simulink model "Battery_sim_2"  (R2026a)
settings: Solver=FixedStepAuto  StopTime=n_years*8760  FixedStep=1
values from neighbouring files (symbols this model uses):
  a_montes = 0.869    [WS_Variables.mat]
  alpha_cal = 0.384    [WS_Variables.mat]
  bpC = [-0.25 -0.2 -0.15 -0.1 -0.05 0 0.05 0.1 0.15 0.2 0.25]    [WS_Variables.mat]
  bpSOC = [0 0.05 0.1 0.15 0.2 0.25 0.3 0.5 0.7 0.75 0.8 0.85 ... (15 elements, 15x1)]    [WS_Variables.mat]
  bpSOH = [0.8 0.9 1]    [WS_Variables.mat]
  dt_h = 1    [WS_Variables.mat]    (also in validate_fixes.m)
  Ea_cal = 20592    [WS_Variables.mat]
  eta_ch = 0.98    [WS_Variables.mat]
  eta_dis = 0.98    [WS_Variables.mat]
  F_const = 96485    [WS_Variables.mat]
  k0_cal = 0.142    [WS_Variables.mat]
  kcal_ref = 0.0003694    [WS_Variables.mat]
  kCch = 0.1038    [WS_Variables.mat]
  kCdch = 0.296    [WS_Variables.mat]
  kcyc = 0.003414    [WS_Variables.mat]
  kDODc = 0.0046    [WS_Variables.mat]
  kmSOC = 0.0513    [WS_Variables.mat]
  kT = 5.8755    [WS_Variables.mat]
  mapCeff = [0 0 0 0 0 0 0.0500000000002 0.1 0.149999999999 0.200000000001 0.249997995467 -0.00299426635782 ... (495 elements, 11x15x3)]    [WS_Variables.mat]
  mapTact = [0 0 0 0 0 0 1.00000000001 1.00000000001 1.00000000001 1.00000000001 1.00000000001 0.414516666666 ... (495 elements, 11x15x3)]    [WS_Variables.mat]
  mSOCref = 0.42    [WS_Variables.mat]
  Q_nom = 3    [WS_Variables.mat]
  R_ch_2D = [0.0536 0.0408 0.0368 0.0344 0.0288 0.0264 0.024 0.0595555555556 0.0453333333333 0.0408888888889 0.0382222222222 0.032 ... (77 elements, 7x11)]    [WS_Variables.mat]
  R_dis_2D = [0.1152 0.088 0.0768 0.072 0.064 0.0576 0.0528 0.0936 0.0715 0.0624 0.0585 0.052 ... (77 elements, 7x11)]    [WS_Variables.mat]
  R_gas = 8.314462618    [WS_Variables.mat]
  SOC0 = 0.5    [WS_Variables.mat]
  SOC_grid = [0 0.1 0.2 0.3 0.4 0.5 0.6 0.7 0.8 0.9 1]    [WS_Variables.mat]
  T_degC = 25    [WS_Variables.mat]
  T_grid_C = [10 20 25 30 40 50 60]    [WS_Variables.mat]
  Tref_cal = 298.15    [WS_Variables.mat]
  Tref_K = 298    [WS_Variables.mat]
  Ua_ref = 0.123    [WS_Variables.mat]
  V_nom = 3.2    [WS_Variables.mat]
undefined symbols (not defined in the file or in its folder): DiscIntNeverNeededParam
libraries: simulink x6
settings Model: Creator=Ali Khedr  LastModifiedBy=diaag
settings SimscapeCC: SimscapeNominalValues="[{\"value\":\"1\",\"unit\":\"A\"},{\"value\":\"1\",\"unit\":\"bar\"},{\"value\":\"1\",\"unit\":\"cm^2\"},{\"value\":\"1\",\"unit\":\"cm^3/s\"},{\"value\":\"1\",\"unit\":\"kJ/kg\"},{\"value\":\"1\",\"unit\":\"kW\"},{\"value\":\"1\",\"unit\":\"l\"},{\"value\":\"1\",\"unit\":\"N\"},{\"value\":\"1\",\"unit\":\"N*m\"},{\"value\":\"1\",\"unit\":\"V\"}]"  SimscapeLogType=none  SimscapeLogDataHistory=5000.0

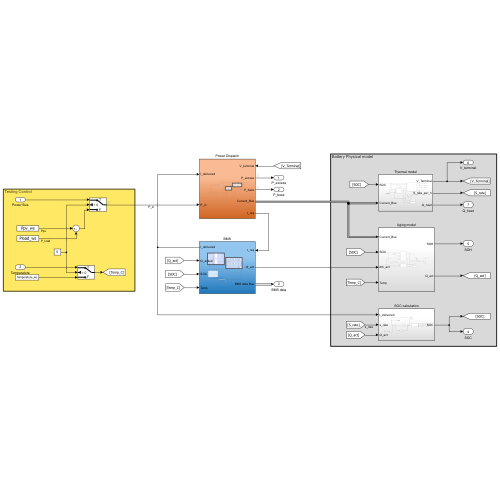
[thumbnail: Simulink's stored preview of the top-level diagram]
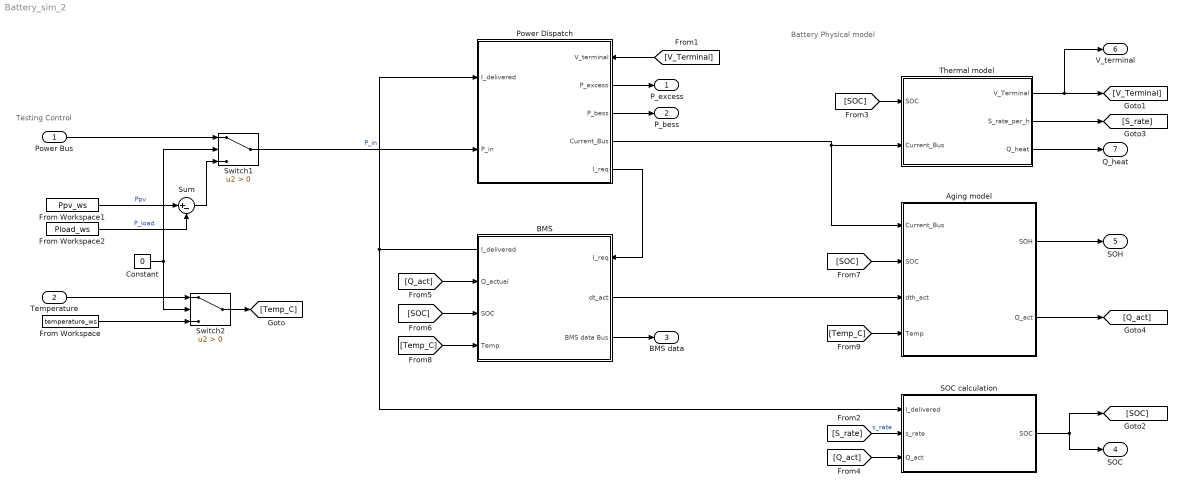
== system Battery_sim_2 ==
  note: Testing Control
  note: Battery Physical model
  Power Bus : Inport
  Temperature : Inport  Port=2
  Aging model : Subsystem
  BMS : Subsystem
      settings: PortSchema="{\"entries\":[{\"content\":{\"sides\":[{\"content\":{\"connectorIds\":[\"In1\",\"Out2\",\"Out3\"]},\"type\":\"ConnectorPlacement.EquallySpacedRectSide\",\"uuid\":\"b0358f3e-70d2-4a9b-a6b5-6f8f3d4044b9\"},{\"content\":{\"connectorIds\":[\"Out1\",\"In2\",\"In3\",\"In4\"],\"side\":\"RIGHT\"},\"type\":\"ConnectorPlacement.EquallySpacedRectSide\",\"uuid\":\"7236fea0-b457-4ecc-99f8-f1352261851b\"},{\"content\":{\"side\":\"TOP\"},\"type\":\"ConnectorPlacement.EquallySpacedRectSide\",\"uuid\":\"a18fdbf6-41d8-4990-8a17-1b53f0b4af4f\"},{\"content\":{\"side\":\"BOTTOM\"},\"type\":\"ConnectorPlacement.EquallySpacedRectSide\",\"uuid\":\"9a35465f-24db-4158-a547-c5af1beda424\"}]},\"type\":\"ConnectorPlacement.EquallySpacedConnector\",\"uuid\":\"ad446661-162d-463d-98d0-534800ba2a51\"}],\"packageUris\":[\"http://schema.mathworks.com/mf0/Connector/R2020b\"],\"version\":\"1.0\"}"
  Constant : Constant  Value=0
  From Workspace : FromWorkspace  VariableName=temperature_ws
  From Workspace1 : FromWorkspace  VariableName=Ppv_ws
  From Workspace2 : FromWorkspace  VariableName=Pload_ws
  Power Dispatch : Subsystem
      settings: PortSchema="{\"entries\":[{\"content\":{\"sides\":[{\"content\":{\"connectorIds\":[\"In1\",\"In2\"]},\"type\":\"ConnectorPlacement.EquallySpacedRectSide\",\"uuid\":\"ee44d7aa-69cc-41bc-9d41-e2128c2b3508\"},{\"content\":{\"connectorIds\":[\"In3\",\"Out1\",\"Out2\",\"Out3\",\"Out4\"],\"side\":\"RIGHT\"},\"type\":\"ConnectorPlacement.EquallySpacedRectSide\",\"uuid\":\"1a9a3f28-b2ae-47b5-968c-66d48cb4930a\"},{\"content\":{\"side\":\"TOP\"},\"type\":\"ConnectorPlacement.EquallySpacedRectSide\",\"uuid\":\"e022eaf0-aade-45fe-ae60-29b950c5dc81\"}]},\"type\":\"ConnectorPlacement.EquallySpacedConnector\",\"uuid\":\"4ff2f9de-87da-4d92-bb97-59c5bfa738bf\"}],\"packageUris\":[\"http://schema.mathworks.com/mf0/Connector/R2020b\"],\"version\":\"1.0\"}"
  SOC calculation : Subsystem
  Sum : Sum  Inputs=|+-
  Switch1 : Switch  Criteria=u2 > Threshold  SaturateOnIntegerOverflow=off  InputSameDT=off
  Switch2 : Switch  Criteria=u2 > Threshold  SaturateOnIntegerOverflow=off  InputSameDT=off
  Thermal model : Subsystem
  P_excess : Outport
  P_bess : Outport  Port=2
  BMS data : Outport  Port=3
  SOC : Outport  Port=4
  SOH : Outport  Port=5
  V_terminal : Outport  Port=6
  Q_heat : Outport  Port=7
  wires:
  Aging model/1(SOH) -> SOH/1
  Aging model/2(Q_act) -> [Q_act]
  [SOC] -> Thermal model/1(SOC)
  Thermal model/1(V_Terminal) -> [V_Terminal], V_terminal/1
  Thermal model/2(S_rate_per_h) -> [S_rate]
  BMS/2(dt_act) -> Aging model/3(dth_act)
  [Q_act] -> BMS/2(Q_actual)
  BMS/1(I_delivered) -> Power Dispatch/1(I_delivered), SOC calculation/1(I_delivered)
  Power Dispatch/3(Current_Bus) -> Aging model/1(Current_Bus), Thermal model/2(Current_Bus)
  [V_Terminal] -> Power Dispatch/3(V_terminal)
  Power Dispatch/4(I_req) -> BMS/1(I_req)
  [S_rate] -> SOC calculation/2(s_rate)  "s_rate"
  [Q_act] -> SOC calculation/3(Q_act)
  SOC calculation/1(SOC) -> SOC/1, [SOC]
  [SOC] -> BMS/3(SOC)
  [Temp_C] -> Aging model/4(Temp)
  [SOC] -> Aging model/2(SOC)
  Power Dispatch/1(P_excess) -> P_excess/1
  Power Dispatch/2(P_bess) -> P_bess/1
  BMS/3(BMS data Bus) -> BMS data/1
  Switch1/1 -> Power Dispatch/2(P_in)  "P_in"
  Constant/1 -> Switch1/2, Switch2/2
  Power Bus/1 -> Switch1/1
  From Workspace2/1 -> Sum/2  "P_load"
  From Workspace1/1 -> Sum/1  "Ppv"
  Sum/1 -> Switch1/3
  From Workspace/1 -> Switch2/3
  Temperature/1 -> Switch2/1
  Switch2/1 -> [Temp_C]
  [Temp_C] -> BMS/4(Temp)
  Thermal model/3(Q_heat) -> Q_heat/1

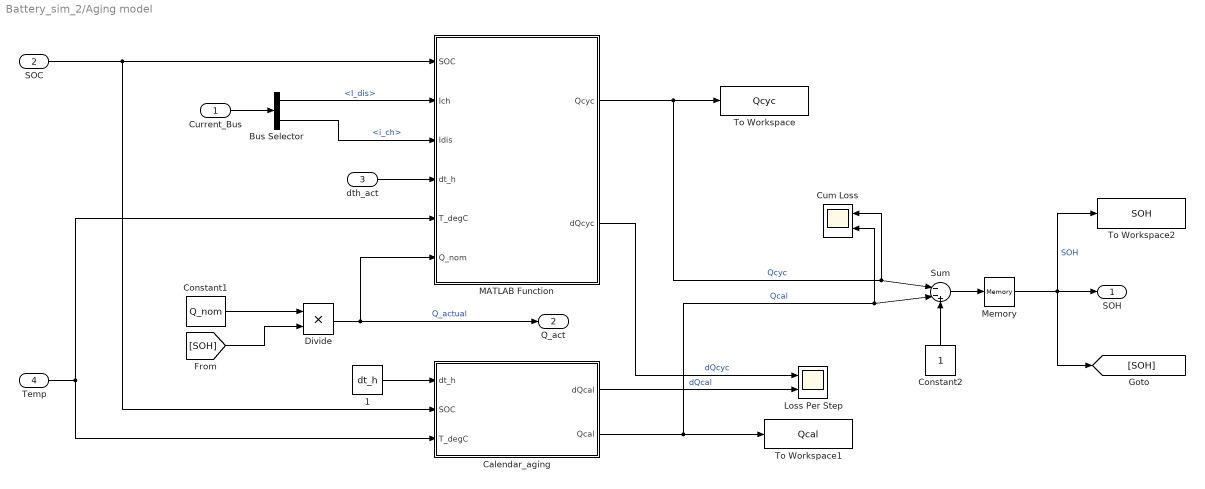
== system Battery_sim_2/Aging model ==
  Current_Bus : Inport
  SOC : Inport  Port=2
  dth_act : Inport  Port=3
  Temp : Inport  Port=4
  " 1" : Constant  Value=dt_h
  Bus Selector : BusSelector  OutputSignals=I_dis,i_ch
  Calendar_aging : Subsystem
  Constant1 : Constant  Value=Q_nom
  Constant2 : Constant
  Cum Loss : Scope  NumInputPorts=2
      settings: ActiveDisplayYMinimum=-0.04665783125845889  ActiveDisplayYMaximum=0.19177623612010322  DataLoggingVariableName=ScopeData5
  Divide : Product  Inputs=**
  Loss Per Step : Scope  NumInputPorts=2
      settings: ActiveDisplayYMinimum=-1.9153240746537514E-5  ActiveDisplayYMaximum=0.00017237916671883764
  MATLAB Function : MATLAB Function  TreatAsAtomicUnit=on
  Memory : Memory  InitialCondition=1
  Sum : Sum  Inputs=|--+
  To Workspace : ToWorkspace  VariableName=Qcyc  SaveFormat=Timeseries  SampleTime=-1
  To Workspace1 : ToWorkspace  VariableName=Qcal  SaveFormat=Timeseries  SampleTime=-1
  To Workspace2 : ToWorkspace  VariableName=SOH  SaveFormat=Timeseries  SampleTime=-1
  SOH : Outport
  Q_act : Outport  Port=2
  wires:
  MATLAB Function/2(dQcyc) -> Loss Per Step/1  "dQcyc"
  Temp/1 -> Calendar_aging/3(T_degC), MATLAB Function/5(T_degC)
  Calendar_aging/2(Qcal) -> To Workspace1/1, Sum/2, Cum Loss/2  "Qcal"
  Constant1/1 -> Divide/1
  Divide/1 -> MATLAB Function/6(Q_nom), Q_act/1  "Q_actual"
  MATLAB Function/1(Qcyc) -> Sum/1, Cum Loss/1, To Workspace/1  "Qcyc"
  Calendar_aging/1(dQcal) -> Loss Per Step/2  "dQcal"
  [SOH] -> Divide/2
  Sum/1 -> Memory/1
  Memory/1 -> [SOH], To Workspace2/1, SOH/1  "SOH"
  Constant2/1 -> Sum/3
  SOC/1 -> MATLAB Function/1(SOC), Calendar_aging/2(SOC)
  dth_act/1 -> MATLAB Function/4(dt_h)
  " 1"/1 -> Calendar_aging/1(dt_h)
  Current_Bus/1 -> Bus Selector/1
  Bus Selector/2 -> MATLAB Function/3(Idis)  "<i_ch>"
  Bus Selector/1 -> MATLAB Function/2(Ich)  "<I_dis>"

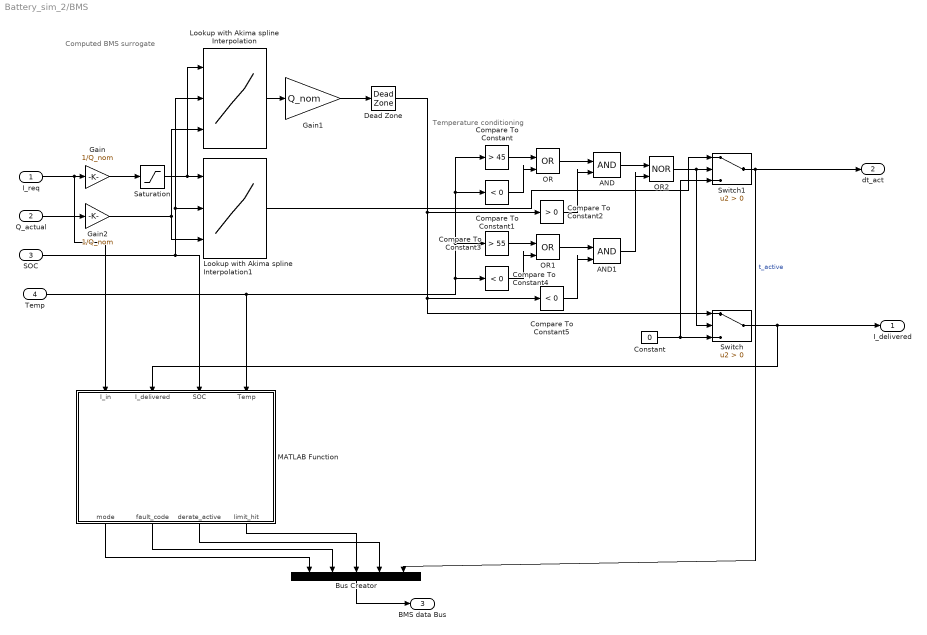
== system Battery_sim_2/BMS ==
  note: Temperature conditioning
  note: Computed BMS surrogate
  I_req : Inport
  Q_actual : Inport  Port=2
  SOC : Inport  Port=3
  Temp : Inport  Port=4
  AND : Logic  IconShape=distinctive  AllPortsSameDT=off  OutDataTypeStr=boolean
  AND1 : Logic  IconShape=distinctive  AllPortsSameDT=off  OutDataTypeStr=boolean
  Bus Creator : BusCreator  Inputs=5  OutDataTypeStr=Bus: BMS_Status  NonVirtualBus=on
      settings: InheritFromInputs=off
  Compare To Constant : simulink/Logic and Bit Operations/Compare To Constant  relop=>  const=45  OutDataTypeStr=boolean
  Compare To Constant1 : simulink/Logic and Bit Operations/Compare To Constant  relop=<  const=0  OutDataTypeStr=boolean
  Compare To Constant2 : simulink/Logic and Bit Operations/Compare To Constant  relop=>  const=0  OutDataTypeStr=boolean
  Compare To Constant3 : simulink/Logic and Bit Operations/Compare To Constant  relop=>  const=55  OutDataTypeStr=boolean
  Compare To Constant4 : simulink/Logic and Bit Operations/Compare To Constant  relop=<  const=0  OutDataTypeStr=boolean
  Compare To Constant5 : simulink/Logic and Bit Operations/Compare To Constant  relop=<  const=0  OutDataTypeStr=boolean
  Constant : Constant  Value=0
  Dead Zone : DeadZone  LowerValue=-0.01  UpperValue=0.0
  Gain : Gain  Gain=1/Q_nom
  Gain1 : Gain  Gain=Q_nom
  Gain2 : Gain  Gain=1/Q_nom
  Lookup with Akima spline Interpolation : Lookup_n-D  NumberOfTableDimensions=3  BreakpointsForDimension1=bpC  BreakpointsForDimension2=bpSOC  BreakpointsForDimension3=bpSOH  BreakpointsForDimension1DataTypeStr=double  BreakpointsForDimension2DataTypeStr=double  BreakpointsForDimension3DataTypeStr=double  Table=mapCeff  TableDataTypeStr=double  IntermediateResultsDataTypeStr=double  InternalRulePriority=Speed  OutDataTypeStr=double  RndMeth=Simplest  FractionDataTypeStr=double  InputSameDT=off
      settings: InputPortMap=u0,u1,u2
  Lookup with Akima spline Interpolation1 : Lookup_n-D  NumberOfTableDimensions=3  BreakpointsForDimension1=bpC  BreakpointsForDimension2=bpSOC  BreakpointsForDimension3=bpSOH  Table=mapTact  InterpMethod=Linear Lagrange  InternalRulePriority=Speed  OutDataTypeStr=double  RndMeth=Simplest
      settings: InputPortMap=u0,u1,u2
  MATLAB Function : MATLAB Function  TreatAsAtomicUnit=on
  OR : Logic  Operator=OR  IconShape=distinctive  AllPortsSameDT=off  OutDataTypeStr=boolean
  OR1 : Logic  Operator=OR  IconShape=distinctive  AllPortsSameDT=off  OutDataTypeStr=boolean
  OR2 : Logic  Operator=NOR  IconShape=distinctive  AllPortsSameDT=off  OutDataTypeStr=boolean
  Saturation : Saturate  UpperLimit=0.25  LowerLimit=-0.25
  Switch : Switch  Criteria=u2 > Threshold  SaturateOnIntegerOverflow=off  InputSameDT=off
  Switch1 : Switch  Criteria=u2 > Threshold  SaturateOnIntegerOverflow=off  InputSameDT=off
  I_delivered : Outport
  dt_act : Outport  Port=2
  BMS data Bus : Outport  Port=3  OutDataTypeStr=Bus: BMS_Status
  wires:
  Compare To Constant/1 -> OR/1
  Compare To Constant1/1 -> OR/2
  Compare To Constant5/1 -> AND1/2
  Compare To Constant4/1 -> OR1/2
  Compare To Constant3/1 -> OR1/1
  OR/1 -> AND/1
  Compare To Constant2/1 -> AND/2
  OR1/1 -> AND1/1
  AND/1 -> OR2/1
  AND1/1 -> OR2/2
  OR2/1 -> Switch1/2, Switch/2
  Constant/1 -> Switch1/3, Switch/3
  Gain/1 -> Saturation/1
  Saturation/1 -> Lookup with Akima spline Interpolation1/1, Lookup with Akima spline Interpolation/1
  Gain2/1 -> Lookup with Akima spline Interpolation/3, Lookup with Akima spline Interpolation1/3
  Gain1/1 -> Dead Zone/1
  Lookup with Akima spline Interpolation/1 -> Gain1/1
  Dead Zone/1 -> Compare To Constant2/1, Compare To Constant5/1, Switch/1
  SOC/1 -> MATLAB Function/3(SOC), Lookup with Akima spline Interpolation/2, Lookup with Akima spline Interpolation1/2
  Temp/1 -> Compare To Constant3/1, Compare To Constant1/1, Compare To Constant/1, Compare To Constant4/1, MATLAB Function/4(Temp)
  Switch1/1 -> Bus Creator/5, dt_act/1  "t_active"
  Lookup with Akima spline Interpolation1/1 -> Switch1/1
  I_req/1 -> MATLAB Function/1(I_in), Gain/1
  Q_actual/1 -> Gain2/1
  Switch/1 -> I_delivered/1, MATLAB Function/2(I_delivered)
  Bus Creator/1 -> BMS data Bus/1
  MATLAB Function/1(mode) -> Bus Creator/1
  MATLAB Function/2(fault_code) -> Bus Creator/2
  MATLAB Function/4(limit_hit) -> Bus Creator/3
  MATLAB Function/3(derate_active) -> Bus Creator/4

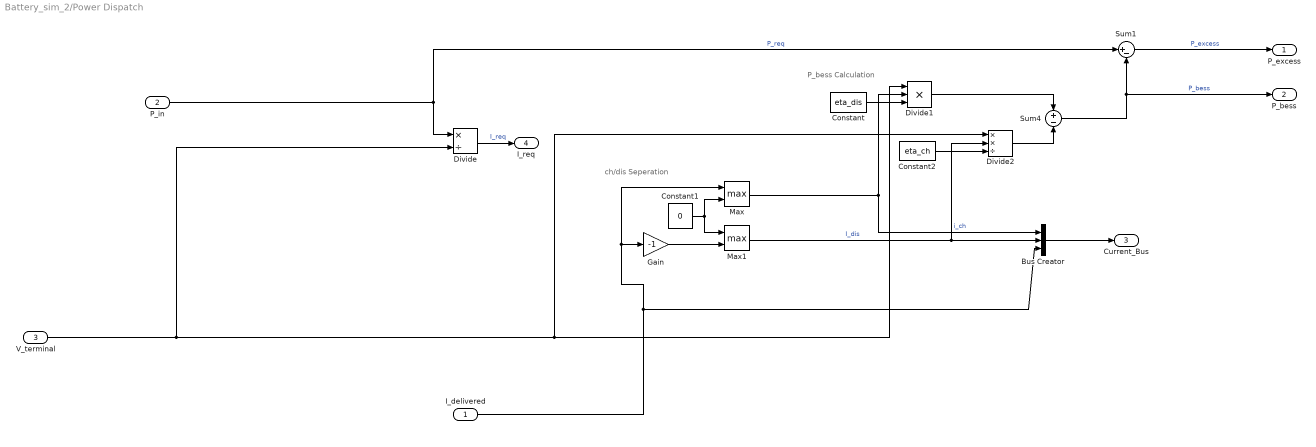
== system Battery_sim_2/Power Dispatch ==
  note: ch/dis Seperation
  note: P_bess Calculation
  I_delivered : Inport
  P_in : Inport  Port=2
  V_terminal : Inport  Port=3
  Bus Creator : BusCreator  Inputs=3
  Constant : Constant  Value=eta_dis
  Constant1 : Constant  Value=0
  Constant2 : Constant  Value=eta_ch
  Divide : Product  Inputs=*/
  Divide1 : Product  Inputs=***
  Divide2 : Product  Inputs=**/
  Gain : Gain  Gain=-1
  Max : MinMax  Function=max  Inputs=2
  Max1 : MinMax  Function=max  Inputs=2
  Sum1 : Sum  Inputs=|+-
  Sum4 : Sum  Inputs=+-
  P_excess : Outport
  P_bess : Outport  Port=2
  Current_Bus : Outport  Port=3
  I_req : Outport  Port=4
  wires:
  Sum4/1 -> Sum1/2, P_bess/1  "P_bess"
  V_terminal/1 -> Divide2/1, Divide1/1, Divide/2
  Max/1 -> Divide1/2, Bus Creator/1  "i_ch"
  Bus Creator/1 -> Current_Bus/1
  Divide2/1 -> Sum4/2
  Gain/1 -> Max1/2
  Divide1/1 -> Sum4/1
  Constant1/1 -> Max/2, Max1/1
  Constant2/1 -> Divide2/3
  Constant/1 -> Divide1/3
  P_in/1 -> Divide/1, Sum1/1  "P_req"
  Max1/1 -> Divide2/2, Bus Creator/2  "I_dis"
  I_delivered/1 -> Max/1, Gain/1, Bus Creator/3
  Divide/1 -> I_req/1  "I_req"
  Sum1/1 -> P_excess/1  "P_excess"

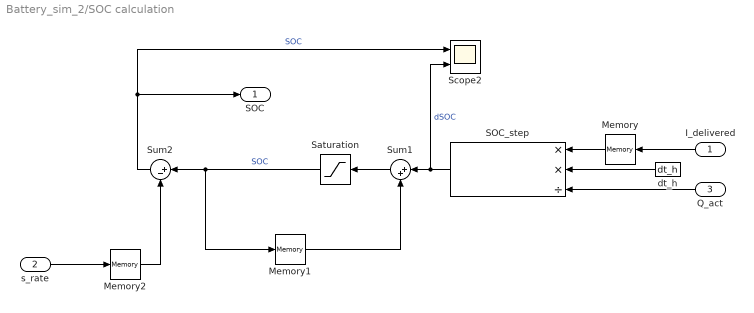
== system Battery_sim_2/SOC calculation ==
  I_delivered : Inport
  s_rate : Inport  Port=2
  Q_act : Inport  Port=3
  Memory : Memory
  Memory1 : Memory  InitialCondition=SOC0
  Memory2 : Memory
  SOC_step : Product  Inputs=**/
  Saturation : Saturate  UpperLimit=1  LowerLimit=0
  Scope2 : Scope  NumInputPorts=2
      settings: ActiveDisplayYMinimum=-0.083070549676689615  ActiveDisplayYMaximum=1.090372335178712  DataLoggingVariableName=ScopeData4
  Sum1 : Sum  Inputs=|++
  Sum2 : Sum  Inputs=|+-
  dt_h : Constant  Value=dt_h
  SOC : Outport
  wires:
  Memory/1 -> SOC_step/1
  Sum2/1 -> SOC/1, Scope2/1  "SOC"
  Memory1/1 -> Sum1/2
  SOC_step/1 -> Sum1/1, Scope2/2  "dSOC"
  Sum1/1 -> Saturation/1
  Saturation/1 -> Memory1/1, Sum2/1  "SOC"
  s_rate/1 -> Memory2/1
  dt_h/1 -> SOC_step/2
  Memory2/1 -> Sum2/2
  Q_act/1 -> SOC_step/3
  I_delivered/1 -> Memory/1

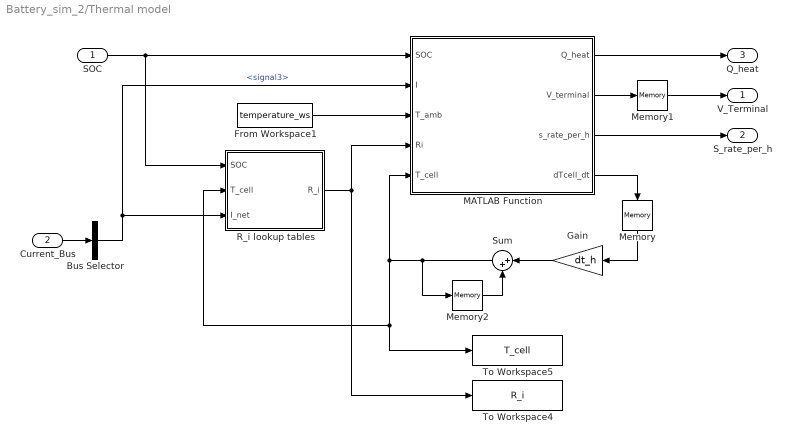
== system Battery_sim_2/Thermal model ==
  SOC : Inport
  Current_Bus : Inport  Port=2
  Bus Selector : BusSelector  OutputSignals=signal3
  From Workspace1 : FromWorkspace  VariableName=temperature_ws
  Gain : Gain  Gain=dt_h
  MATLAB Function : MATLAB Function  TreatAsAtomicUnit=on
  Memory : Memory
  Memory1 : Memory  InitialCondition=V_nom
  Memory2 : Memory  InitialCondition=T_degC
  R_i lookup tables : Subsystem
  Sum : Sum  Inputs=|++
  To Workspace4 : ToWorkspace  VariableName=R_i  SaveFormat=Timeseries  SampleTime=-1
  To Workspace5 : ToWorkspace  VariableName=T_cell  SaveFormat=Timeseries  SampleTime=-1
  V_Terminal : Outport
  S_rate_per_h : Outport  Port=2
  Q_heat : Outport  Port=3
  wires:
  Current_Bus/1 -> Bus Selector/1
  SOC/1 -> R_i lookup tables/1(SOC), MATLAB Function/1(SOC)
  From Workspace1/1 -> MATLAB Function/3(T_amb)
  MATLAB Function/2(V_terminal) -> Memory1/1
  MATLAB Function/4(dTcell_dt) -> Memory/1
  Memory/1 -> Gain/1
  Sum/1 -> To Workspace5/1, R_i lookup tables/2(T_cell), MATLAB Function/5(T_cell), Memory2/1
  Gain/1 -> Sum/1
  Memory2/1 -> Sum/2
  MATLAB Function/3(s_rate_per_h) -> S_rate_per_h/1
  R_i lookup tables/1(R_i) -> MATLAB Function/4(Ri), To Workspace4/1
  Memory1/1 -> V_Terminal/1
  Bus Selector/1 -> MATLAB Function/2(I), R_i lookup tables/3(I_net)  "<signal3>"
  MATLAB Function/1(Q_heat) -> Q_heat/1

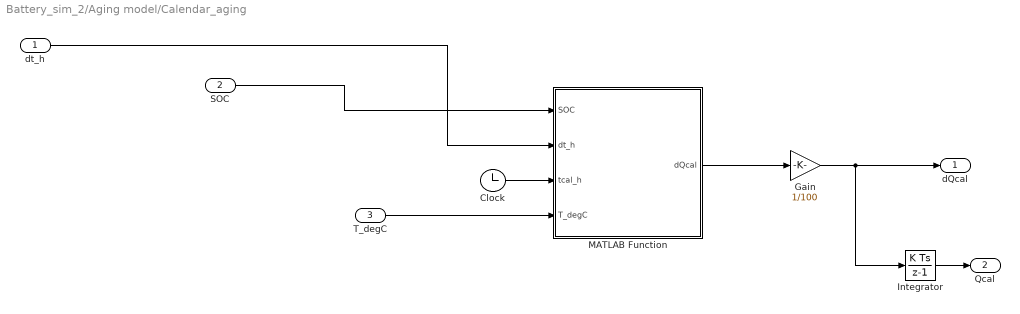
== system Battery_sim_2/Aging model/Calendar_aging ==
  dt_h : Inport
  SOC : Inport  Port=2
  T_degC : Inport  Port=3
  Clock : Clock
  Gain : Gain  Gain=1/100
  Integrator : DiscreteIntegrator  ICPrevOutput=DiscIntNeverNeededParam  ICPrevScaledInput=DiscIntNeverNeededParam
  MATLAB Function : MATLAB Function  TreatAsAtomicUnit=on
  dQcal : Outport
  Qcal : Outport  Port=2
  wires:
  SOC/1 -> MATLAB Function/1(SOC)
  Clock/1 -> MATLAB Function/3(tcal_h)
  dt_h/1 -> MATLAB Function/2(dt_h)
  MATLAB Function/1(dQcal) -> Gain/1
  T_degC/1 -> MATLAB Function/4(T_degC)
  Gain/1 -> dQcal/1, Integrator/1
  Integrator/1 -> Qcal/1

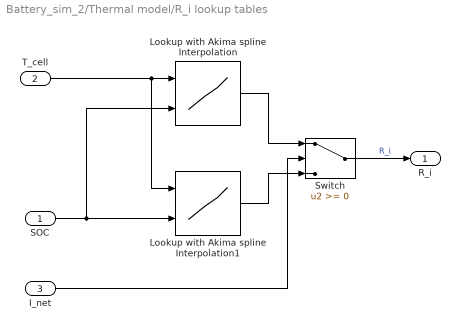
== system Battery_sim_2/Thermal model/R_i lookup tables ==
  SOC : Inport
  T_cell : Inport  Port=2
  I_net : Inport  Port=3
  Lookup with Akima spline Interpolation : Lookup_n-D  BreakpointsForDimension1=T_grid_C  BreakpointsForDimension2=SOC_grid  Table=R_ch_2D  InterpMethod=Akima spline  InternalRulePriority=Speed  RndMeth=Simplest
      settings: InputPortMap=u0,u1
  Lookup with Akima spline Interpolation1 : Lookup_n-D  BreakpointsForDimension1=T_grid_C  BreakpointsForDimension2=SOC_grid  Table=R_dis_2D  InterpMethod=Akima spline  InternalRulePriority=Speed  RndMeth=Simplest
      settings: InputPortMap=u0,u1
  Switch : Switch  SaturateOnIntegerOverflow=off  InputSameDT=off
  R_i : Outport
  wires:
  Lookup with Akima spline Interpolation/1 -> Switch/1
  Switch/1 -> R_i/1  "R_i"
  SOC/1 -> Lookup with Akima spline Interpolation/2, Lookup with Akima spline Interpolation1/2
  Lookup with Akima spline Interpolation1/1 -> Switch/3
  I_net/1 -> Switch/2
  T_cell/1 -> Lookup with Akima spline Interpolation1/1, Lookup with Akima spline Interpolation/1

== matlab function Battery_sim_2/Aging model/Calendar_aging/MATLAB Function ==
  data: SOC input; dQcal output; dt_h input; tcal_h input; T_degC input; Ea_cal parameter; R_gas parameter; Tref_cal parameter; alpha_cal parameter; F_const parameter; Ua_ref parameter; k0_cal parameter; kcal_ref parameter
function dQcal = calendar_aging(SOC, dt_h, tcal_h, T_degC, ...
    Ea_cal, R_gas, Tref_cal, alpha_cal, F_const, Ua_ref, k0_cal, kcal_ref)

dQcal = calendar_aging(SOC, dt_h, tcal_h, T_degC, ...
    Ea_cal, R_gas, Tref_cal, alpha_cal, F_const, Ua_ref, k0_cal, kcal_ref);
end

== matlab function Battery_sim_2/BMS/MATLAB Function ==
  settings: updateMethod=DISCRETE
  data: I_in input; I_delivered input; SOC input; mode output; Temp input; fault_code output; derate_active output boolean; limit_hit output
function [mode, fault_code, derate_active, limit_hit] = bms_status(I_in, I_delivered, SOC, Temp)
  cfg = bms_config();
  idle = cfg.mode.I_idle_thr;

  charging    = I_delivered >  idle;
  discharging = I_delivered < -idle;

  reduced = abs(I_delivered) < abs(I_in) - idle;          % limited but flowing
  cut     = (abs(I_in) > idle) && (abs(I_delivered) <= idle);  % fully blocked

  % why it was blocked (instantaneous, no latch)
  cold  = (Temp < cfg.cell.T_chg_min);
  hot   = (charging && Temp > cfg.cell.T_chg_max) || (discharging && Temp > cfg.cell.T_dis_max);
  soclim = (charging && SOC >= cfg.soc.window_max) || (discharging && SOC <= cfg.soc.window_min);

  fault_code = 0;                       % 0 none
  if cut
      if cold,  fault_code = 1;         % cold-charge block
      elseif hot, fault_code = 2;       % over-temp block
      elseif soclim, fault_code = 3;    % SOC floor/ceiling
      else 
          fault_code = 4; end          % other (request cut for another reason)
  end

  derate_active = reduced && ~cut;
  limit_hit     = cut;

  if cut,               mode = cfg.mode.FAULT;
  elseif derate_active, mode = cfg.mode.DERATE;
  elseif charging,      mode = cfg.mode.CHARGE;
  elseif discharging,   mode = cfg.mode.DISCHARGE;
  else                  mode = cfg.mode.STANDBY;
  end
end

== matlab function Battery_sim_2/Aging model/MATLAB Function ==
  settings: updateMethod=DISCRETE
  data: SOC input; Qcyc output; Ich input; Idis input; dt_h input; T_degC input; Q_nom input; kT parameter; Tref_K parameter; kDODc parameter; kcyc parameter; kCch parameter; kCdch parameter; kmSOC parameter; mSOCref parameter; a_montes parameter; dQcyc output
function [Qcyc, dQcyc] = cycle_aging(SOC, Ich, Idis, dt_h, T_degC, Q_nom, ...
    kT, Tref_K, kDODc, kcyc, kCch, kCdch, kmSOC, mSOCref, a_montes)

[Qcyc, dQcyc] = cycle_aging(SOC, Ich, Idis, dt_h, T_degC, Q_nom, ...
    kT, Tref_K, kDODc, kcyc, kCch, kCdch, kmSOC, mSOCref, a_montes);

Qcyc = Qcyc / 100;
dQcyc = dQcyc / 100;

end

== matlab function Battery_sim_2/Thermal model/MATLAB Function ==
  data: SOC input; I input; T_amb input; Q_heat output; V_terminal output; s_rate_per_h output; dTcell_dt output; Ri input; T_cell input
function [Q_heat, V_terminal, s_rate_per_h, dTcell_dt] = cell_thermal(SOC, I,T_amb,Ri, T_cell)

  [Q_heat, V_terminal, s_rate_per_h, dTcell_dt] = cell_thermal(SOC, I,T_cell, T_amb,Ri);

end
